simulink model "ADRCControl_CDPR_6DOF_20220708"  (R2020a)
settings: Solver=VariableStepAuto  StartTime=0.0  StopTime=12  RelTol=1e-3  EnableMultiTasking=on
values from neighbouring files (symbols this model uses):
  a = 25    [parameters_initialization.m]
  b = 0.05    [parameters_initialization.m]
  Kd = 7.062    [parameters_initialization.m]
  Kp = 70    [parameters_initialization.m]
undefined symbols (not defined in the file or in its folder): X, Y, Z
libraries: sm_lib x150, nesl_utility x52, sm_cable_robot_lib x30, simulink x1
(part 8 of 8)

== system ADRCControl_CDPR_6DOF_20220708/6DOF CDPR/Subsystem/3/Motor Assembly2/Motor ==
  Flange : sm_lib/Body Elements/Cylindrical Solid  GraphicAmbientColor=[0.15 0.15 0.15 1.0]  BasedOnType=Density  CenterOfMass=[0 0 0]  CenterOfMassUnits=m  GraphicDiffuseColor=flangeColor  CylinderLength=flangeThickness  CylinderLengthUnits=m  CylinderRadius=flangeRadius  CylinderRadiusUnits=m  Density=housingRho  DensityUnits=kg/m^3  DoExposeReferenceFrame=off  GraphicEmissiveColor=[0.0 0.0 0.0 1.0]  ExportEntireGeometry=off  SerializedFrames=<Frames><Frame><Id>Frame1</Id><Value><Name>B</Name><Origin><Source>GeometricFeature</Source><FeatureName>bottom surface</FeatureName></Origin><PrimaryAxis><DefinedDirection>+Z</DefinedDirection><Source>ReferenceFrame</Source><SourceDirection>+Z</SourceDirection><FeatureName></FeatureName></PrimaryAxis><SecondaryAxis><DefinedDirection>+X</DefinedDirection><Source>ReferenceFrame</Source><SourceDirection>+X</SourceDirection><FeatureName></FeatureName></SecondaryAxis></Value></Frame></Frames>  MarkerShape=Sphere  MarkerSize=10  GraphicType=FromGeometry  InertiaType=CalculateFromGeometry  Mass=1  MassUnits=kg  MomentsOfInertia=[1 1 1]  MomentsOfInertiaUnits=kg*m^2  GraphicOpacity=1.0  ProductsOfInertia=[0 0 0]  ProductsOfInertiaUnits=kg*m^2  GraphicShininess=75  GraphicSpecularColor=[0.5 0.5 0.5 1.0]  GraphicVisPropType=SimpleVisualProperties
  Housing : sm_lib/Body Elements/Brick Solid  GraphicAmbientColor=[0.15 0.15 0.15 1.0]  BasedOnType=Density  BrickDimensions=[width height depth]  BrickDimensionUnits=m  CenterOfMass=[0 0 0]  CenterOfMassUnits=m  GraphicDiffuseColor=housingColor  Density=housingRho  DensityUnits=kg/m^3  DoExposeReferenceFrame=off  GraphicEmissiveColor=[0.0 0.0 0.0 1.0]  ExportEntireGeometry=off  SerializedFrames=<Frames><Frame><Id>Frame2</Id><Value><Name>B</Name><Origin><Source>GeometricFeature</Source><FeatureName>+x -y +z point</FeatureName></Origin><PrimaryAxis><DefinedDirection>+Z</DefinedDirection><Source>ReferenceFrame</Source><SourceDirection>+Z</SourceDirection><FeatureName></FeatureName></PrimaryAxis><SecondaryAxis><DefinedDirection>+X</DefinedDirection><Source>ReferenceFrame</Source><SourceDirection>+X</SourceDirection><FeatureName></FeatureName></SecondaryAxis></Value></Frame><Frame><Id>Frame3</Id><Value><Name>F</Name><Origin><Source>GeometricFeature</Source><FeatureName>+z surface</FeatureName></Origin><PrimaryAxis><DefinedDirection>+Z</DefinedDirection><Source>ReferenceFrame</Source><SourceDirection>+Z</SourceDirection><FeatureName></FeatureName></PrimaryAxis><SecondaryAxis><DefinedDirection>+X</DefinedDirection><Source>ReferenceFrame</Source><SourceDirection>+X</SourceDirection><FeatureName></FeatureName></SecondaryAxis></Value></Frame></Frames>  MarkerShape=Sphere  MarkerSize=10  GraphicType=FromGeometry  InertiaType=CalculateFromGeometry  Mass=1  MassUnits=kg  MomentsOfInertia=[1 1 1]  MomentsOfInertiaUnits=kg*m^2  GraphicOpacity=1.0  ProductsOfInertia=[0 0 0]  ProductsOfInertiaUnits=kg*m^2  GraphicShininess=75  GraphicSpecularColor=[0.5 0.5 0.5 1.0]  GraphicVisPropType=SimpleVisualProperties
  Motor Revolute : sm_lib/Joints/Revolute Joint  JointMode=Normal  SenseConstraintForce=off  SenseConstraintForceX=off  SenseConstraintForceY=off  SenseConstraintForceZ=off  SenseConstraintTorque=off  SenseConstraintTorqueX=off  SenseConstraintTorqueY=off  SenseConstraintTorqueZ=off  SenseTotalForce=off  SenseTotalForceX=off  SenseTotalForceY=off  SenseTotalForceZ=off  SenseTotalTorque=off  SenseTotalTorqueX=off  SenseTotalTorqueY=off  SenseTotalTorqueZ=off  CompositeWrenchDir=FollowerOnBase  CompositeWrenchFrame=BaseFrame  EquilibriumPosition=0  EquilibriumPositionUnits=deg  SpringStiffness=0  SpringStiffnessUnits=N*m/deg  DampingCoefficient=0  DampingCoefficientUnits=N*m/(deg/s)  TorqueActuationMode=InputTorque  MotionActuationMode=ComputedMotion  SensePosition=on  SenseVelocity=off  SenseAcceleration=off  SenseTorqueForce=on  SenseLowerLimitTorqueForce=off  SenseUpperLimitTorqueForce=off  LowerLimitSpecify=off  LowerLimitBound=-90  LowerLimitBoundUnits=deg  LowerLimitStiffness=1e4  LowerLimitStiffnessUnits=N*m/deg  LowerLimitDamping=10  LowerLimitDampingUnits=N*m/(deg/s)  LowerLimitTransitionRegionWidth=0.1  LowerLimitTransitionRegionWidthUnits=deg  UpperLimitSpecify=off  UpperLimitBound=90  UpperLimitBoundUnits=deg  UpperLimitStiffness=1e4  UpperLimitStiffnessUnits=N*m/deg  UpperLimitDamping=10  UpperLimitDampingUnits=N*m/(deg/s)  UpperLimitTransitionRegionWidth=0.1  UpperLimitTransitionRegionWidthUnits=deg  PositionTargetSpecify=off  PositionTargetPriority=High  PositionTargetValue=0  PositionTargetValueUnits=deg  VelocityTargetSpecify=off  VelocityTargetPriority=High  VelocityTargetValue=0  VelocityTargetValueUnits=deg/s
  PS-Simulink Converter1 : nesl_utility/PS-Simulink Converter  PhysicalDomain=network_engine_domain  SubClassName=ps_output  LeftPortType=input  RightPortType=output  PseudoPeriodic=off  Frequencies=[]  Unit=inherit  AffineConversion=off
  PS-Simulink Converter10 : nesl_utility/PS-Simulink Converter  PhysicalDomain=network_engine_domain  SubClassName=ps_output  LeftPortType=input  RightPortType=output  PseudoPeriodic=off  Frequencies=[]  Unit=inherit  AffineConversion=off
  Shaft : sm_lib/Body Elements/Cylindrical Solid  GraphicAmbientColor=[0.15 0.15 0.15 1.0]  BasedOnType=Density  CenterOfMass=[0 0 0]  CenterOfMassUnits=m  GraphicDiffuseColor=shaftColor  CylinderLength=shaftLength  CylinderLengthUnits=m  CylinderRadius=shaftRadius  CylinderRadiusUnits=m  Density=shaftRho  DensityUnits=kg/m^3  DoExposeReferenceFrame=on  GraphicEmissiveColor=[0.0 0.0 0.0 1.0]  ExportEntireGeometry=off  SerializedFrames=<Frames><Frame><Id>Frame1</Id><Value><Name>B</Name><Origin><Source>GeometricFeature</Source><FeatureName>bottom surface</FeatureName></Origin><PrimaryAxis><DefinedDirection>+Z</DefinedDirection><Source>ReferenceFrame</Source><SourceDirection>+Z</SourceDirection><FeatureName></FeatureName></PrimaryAxis><SecondaryAxis><DefinedDirection>+X</DefinedDirection><Source>ReferenceFrame</Source><SourceDirection>+X</SourceDirection><FeatureName></FeatureName></SecondaryAxis></Value></Frame></Frames>  MarkerShape=Sphere  MarkerSize=10  GraphicType=FromGeometry  InertiaType=CalculateFromGeometry  Mass=1  MassUnits=kg  MomentsOfInertia=[1 1 1]  MomentsOfInertiaUnits=kg*m^2  GraphicOpacity=1.0  ProductsOfInertia=[0 0 0]  ProductsOfInertiaUnits=kg*m^2  GraphicShininess=75  GraphicSpecularColor=[0.5 0.5 0.5 1.0]  GraphicVisPropType=SimpleVisualProperties
  Simulink-PS Converter : nesl_utility/Simulink-PS Converter  PhysicalDomain=network_engine_domain  SubClassName=ps_input  LeftPortType=input  RightPortType=output  PseudoPeriodic=off  Frequencies=[]  NoiseDistribution=none  NoiseParameters=[]  Unit=N*m  AffineConversion=off  FilteringAndDerivatives=filter  SimscapeFilterOrder=2  InputFilterTimeConstant=0.001  UdotUserProvided=0
  Sum1 : Sum  Inputs=+-
  B : PMIOPort  Side=Left
  S : PMIOPort  Port=2  Side=Right
  tag scope: C2Mq=global, C2Mtrq=global
  wires:
  PS-Simulink Converter10/1 -> [C2Mtrq]
  [C2Intrq] -> Sum1/1
  [C2Outtrq] -> Sum1/2
  PS-Simulink Converter1/1 -> [C2Mq]
  Sum1/1 -> Simulink-PS Converter/1
  connections:
  Housing/LConn1 -- B/RConn1
  S/RConn1 -- Shaft/RConn1
  Shaft/LConn1 -- Motor Revolute/RConn1
  Flange/LConn1 -- Housing/RConn1 -- Motor Revolute/LConn1
  Motor Revolute/LConn2 -- Simulink-PS Converter/RConn1
  PS-Simulink Converter10/LConn1 -- Motor Revolute/RConn3
  PS-Simulink Converter1/LConn1 -- Motor Revolute/RConn2

== matlab function ADRCControl_CDPR_6DOF_20220708/ADRC Torque Controller/2-Order ADRC Contoller1 /ESO parameters assignment ==
  data: omega input; beta01 output; beta02 output; beta03 output
function [beta01,beta02,beta03] = fcn(omega)
    beta01 = 3*omega;
    beta02 = 3/5*omega^2;
    beta03 = 1/9*omega^3;
end

== matlab function ADRCControl_CDPR_6DOF_20220708/Desired Intput Signal/Desried Angle ==
  data: t input; A1q output; A2q output; B1q output; B2q output; C1q output; C2q output
function [A1q,A2q,B1q,B2q,C1q,C2q] = fcn(t)

A1q = - 5.073*sin(0.5272*t - 2.628 ) - 18.79*sin(0.0022*t + 0.1229);
A2q =  5.073*sin(0.5272*t - 2.628 ) + 18.79*sin(0.0022*t + 0.1229);
B1q = - 7.131*sin(0.1979*t - 2.758) - 3.267*sin(0.623*t + 0.9728);
B2q = 7.131*sin(0.1979*t - 2.758) + 3.267*sin(0.623*t + 0.9728);
C1q = -5.081*sin(0.5266*t - 0.5543) - 23.91*sin(0.001593*t + 3.025);
C2q = 5.081*sin(0.5266*t - 0.5543) + 23.91*sin(0.001593*t + 3.025);

end

== matlab function ADRCControl_CDPR_6DOF_20220708/ADRC Torque Controller/2-Order ADRC Contoller2/ESO parameters assignment ==
  data: omega input; beta01 output; beta02 output; beta03 output
function [beta01,beta02,beta03] = fcn(omega)
    beta01 = 3*omega;
    beta02 = 3/5*omega^2;
    beta03 = 1/9*omega^3;
end

== matlab function ADRCControl_CDPR_6DOF_20220708/ADRC Torque Controller/2-Order ADRC Contoller3/ESO parameters assignment ==
  data: omega input; beta01 output; beta02 output; beta03 output
function [beta01,beta02,beta03] = fcn(omega)
    beta01 = 3*omega;
    beta02 = 3/5*omega^2;
    beta03 = 1/9*omega^3;
end

== matlab function ADRCControl_CDPR_6DOF_20220708/ADRC Torque Controller/2-Order ADRC Contoller4/ESO parameters assignment ==
  data: omega input; beta01 output; beta02 output; beta03 output
function [beta01,beta02,beta03] = fcn(omega)
    beta01 = 3*omega;
    beta02 = 3/5*omega^2;
    beta03 = 1/9*omega^3;
end

== matlab function ADRCControl_CDPR_6DOF_20220708/ADRC Torque Controller/2-Order ADRC Contoller_5/ESO parameters assignment ==
  data: omega input; beta01 output; beta02 output; beta03 output
function [beta01,beta02,beta03] = fcn(omega)
    beta01 = 3*omega;
    beta02 = 3/5*omega^2;
    beta03 = 1/9*omega^3;
end

== matlab function ADRCControl_CDPR_6DOF_20220708/ADRC Torque Controller/2-Order ADRC Contoller6/ESO parameters assignment ==
  data: omega input; beta01 output; beta02 output; beta03 output
function [beta01,beta02,beta03] = fcn(omega)
    beta01 = 3*omega;
    beta02 = 3/5*omega^2;
    beta03 = 1/9*omega^3;
end

== matlab function ADRCControl_CDPR_6DOF_20220708/Desired Intput Signal/Desried Torque1 ==
  data: t input; A1q output; A2q output; B1q output; B2q output; C1q output; C2q output
function [A1q,A2q,B1q,B2q,C1q,C2q] = fcn(t)

A1q = -2.719 *sin(0.5221*t - 1.041);
A2q = 2.719 *sin(0.5221*t - 1.041);
B1q = -2.747 *sin(0.5328*t + 3.085);
B2q = 2.747 *sin(0.5328*t + 3.085);
C1q = -2.718*sin(0.5231*t + 1.048);
C2q = 2.718*sin(0.5231*t + 1.048);

end
